simulink model "Encoder_Sensor"  (R2018a)
settings: Solver=VariableStepAuto  StartTime=0.0  StopTime=10.0  RelTol=1e-3
PreLoadFcn:
  | modelDir = fileparts(get_param(bdroot, 'FileName'));
  | addpath(fullfile(modelDir,'Parameters'));
  | addpath(fullfile(modelDir,'subsystems'));
  | 
  | Parameters_Model
  | Parameters_Simulation
  | Parameters_Estimators
InitFcn:
  | Parameters_Model
  | Parameters_Simulation
  | Parameters_Estimators
undefined symbols (not defined in the file): EnableNoise, sensor_sigma2_encoder, TicksPrRev, Ts_encoder
settings Model: Creator=Thomas  LastModifiedBy=Thomas

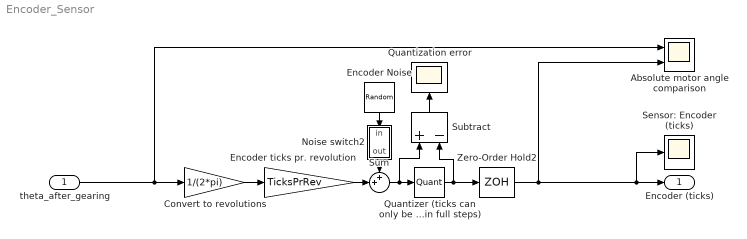
== system Encoder_Sensor ==
  theta_after_gearing : Inport
  Absolute motor angle comparison : Scope  NumInputPorts=2
  Convert to revolutions : Gain  Gain=1/(2*pi)
  Encoder Noise : RandomNumber  Variance=sensor_sigma2_encoder  Seed=81  SampleTime=Ts_encoder
  Encoder ticks pr. revolution : Gain  Gain=TicksPrRev
  Noise switch2 : Subsystem
  Quantization error : Scope
  Quantizer (ticks can only be measured in full steps) : Quantizer  QuantizationInterval=1
  Sensor: Encoder (ticks) : Scope
  Subtract : Sum  Inputs=+-
  Sum : Sum  Inputs=++|
  Zero-Order Hold2 : ZeroOrderHold  SampleTime=Ts_encoder
  Encoder (ticks) : Outport
  wires:
  Zero-Order Hold2/1 -> Absolute motor angle comparison/2, Encoder (ticks)/1, Sensor: Encoder (ticks)/1
  theta_after_gearing/1 -> Absolute motor angle comparison/1, Convert to revolutions/1
  Sum/1 -> Subtract/1, Quantizer (ticks can only be measured in full steps)/1
  Encoder Noise/1 -> Noise switch2/1(in)
  Encoder ticks pr. revolution/1 -> Sum/2
  Convert to revolutions/1 -> Encoder ticks pr. revolution/1
  Subtract/1 -> Quantization error/1
  Noise switch2/1(out) -> Sum/1
  Quantizer (ticks can only be measured in full steps)/1 -> Subtract/2, Zero-Order Hold2/1

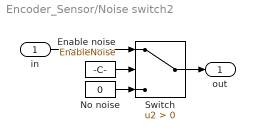
== system Encoder_Sensor/Noise switch2 ==
  in : Inport
  Enable noise : Constant  Value=EnableNoise
  No noise : Constant  Value=0
  Switch : Switch  Criteria=u2 > Threshold
  out : Outport
  wires:
  No noise/1 -> Switch/3
  Switch/1 -> out/1
  Enable noise/1 -> Switch/2
  in/1 -> Switch/1
